simulink model "DualIFreciever"  (R2015b)
settings: Solver=FixedStepAuto  StartTime=0.0  StopTime=0.01  SampleTimeConstraint=Specified
libraries: rfmathmodels1 x8, commrflib2 x1, dspxfrm3 x1, dspvision x1, commanabbnd3 x1
settings Model: Creator=dominikguz  LastModifiedBy=dominikguz

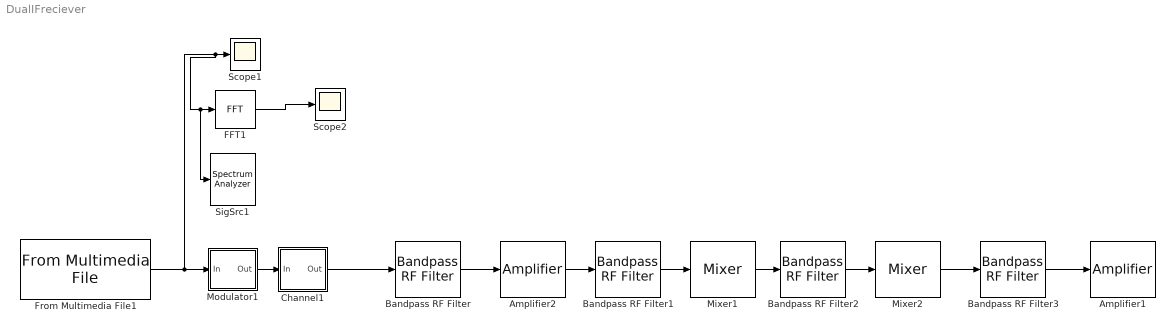
== system DualIFreciever ==
  Amplifier1 : rfmathmodels1/Amplifier  model_select=Linear  linGaindB=0  GindB=0  iip3=30  am2pm=10  PwrAMPMStart=10  PwrAMPMEnd=inf  amam=[2.1587 1.1517]  ampm=[4.0033 9.1040]  x=[8.1081 1.5413 6.5202 -0.0718]  y=[4.6645 2.0965 10.88 -0.003]  p=0.5  GoutdB=0  vsat=1  method_select=Noise factor  ntemp=290  nfigure=3.01  nfactor=2  seed=67987
  Amplifier2 : rfmathmodels1/Amplifier  model_select=Linear  linGaindB=0  GindB=0  iip3=30  am2pm=10  PwrAMPMStart=10  PwrAMPMEnd=inf  amam=[2.1587 1.1517]  ampm=[4.0033 9.1040]  x=[8.1081 1.5413 6.5202 -0.0718]  y=[4.6645 2.0965 10.88 -0.003]  p=0.5  GoutdB=0  vsat=1  method_select=Noise factor  ntemp=290  nfigure=3.01  nfactor=2  seed=67987
  Bandpass RF Filter{,1..3} (4 alike) : rfmathmodels1/Bandpass RF Filter  method=Butterworth  filttype=Bandpass  N=3  flo=1.9998e9  fhi=2.0002e9  Rp=1  Rs=10  MaxLength=32  Fc=2e9  Ts=1e-6
  Channel1 : Subsystem
  FFT1 : dspxfrm3/FFT  FFTImplementation=Auto  CompMethod=Table lookup  TableOpt=NEW  TableOptActive=Speed  BitRevOrder=off  Normalize=off  InheritFFTLength=on  FFTLength=64  WrapInput=on  roundingMode=Floor  overflowMode=off  firstCoeffDataTypeStr=Inherit: Same word length as input  firstCoeffLastDataTypeStr=Inherit: Same word length as input  outputMin=[]  outputMax=[]
  From Multimedia File1 : dspvision/From Multimedia File  inputFilename=guitartune.wav  loop=on  numPlays=1  outputStreams=Audio only  videoDataType=single  audioDataType=double  inheritSampleTime=on  userDefinedSampleTime=1/4410  noAudioOutput=off  isIntensityVideo=off  fourcc=RGB  colorVideoFormat=Separate color signals  outputEOF=off  dataOrg=Column-major  audioFrameSize=4410  computeAudioFrameSize=off  outSamplingMode=Sample based
  Mixer1 : rfmathmodels1/Mixer  gain=0  PhNs=-120  Fo=100  seed=2137  loss=0
  Mixer2 : rfmathmodels1/Mixer  gain=0  PhNs=-120  Fo=100  seed=2137  loss=0
  Modulator1 : Subsystem
  Scope1 : Scope
  Scope2 : Scope
  SigSrc1 : SpectrumAnalyzer
  wires:
  Bandpass RF Filter1/1 -> Mixer1/1
  Mixer1/1 -> Bandpass RF Filter2/1
  Bandpass RF Filter/1 -> Amplifier2/1
  Bandpass RF Filter3/1 -> Amplifier1/1
  Amplifier2/1 -> Bandpass RF Filter1/1
  Bandpass RF Filter2/1 -> Mixer2/1
  Mixer2/1 -> Bandpass RF Filter3/1
  Modulator1/1(Out) -> Channel1/1(In)
  Channel1/1(Out) -> Bandpass RF Filter/1
  From Multimedia File1/1 -> SigSrc1/1, FFT1/1, Scope1/1, Modulator1/1(In)
  FFT1/1 -> Scope2/1

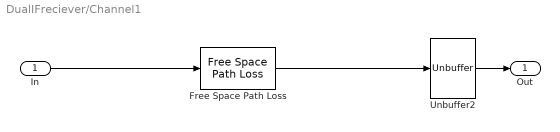
== system DualIFreciever/Channel1 ==
  In : Inport
  Free Space Path Loss : commrflib2/Free Space Path Loss  mode=Decibels  dB=120  d=0.100  fc=1920
  Unbuffer2 : Unbuffer  SampleBasedProcessing=Same as frame based
  Out : Outport
  wires:
  Free Space Path Loss/1 -> Unbuffer2/1
  Unbuffer2/1 -> Out/1
  In/1 -> Free Space Path Loss/1

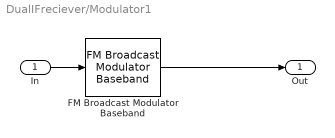
== system DualIFreciever/Modulator1 ==
  In : Inport
  FM Broadcast Modulator Baseband : commanabbnd3/FM Broadcast Modulator Baseband  SampleRate=152e3  FrequencyDeviation=75e3  FilterTimeConstant=75e-6  AudioSampleRate=44100  Stereo=off  SimulateUsing=Code generation
  Out : Outport
  wires:
  In/1 -> FM Broadcast Modulator Baseband/1
  FM Broadcast Modulator Baseband/1 -> Out/1
